simulink model "dcMotor_DiagramBlocks"  (R2018a)
settings: Solver=VariableStepAuto  StartTime=0.0  StopTime=10.0  RelTol=1e-3
libraries: simulink x4
settings Model: Creator=Igor  LastModifiedBy=david

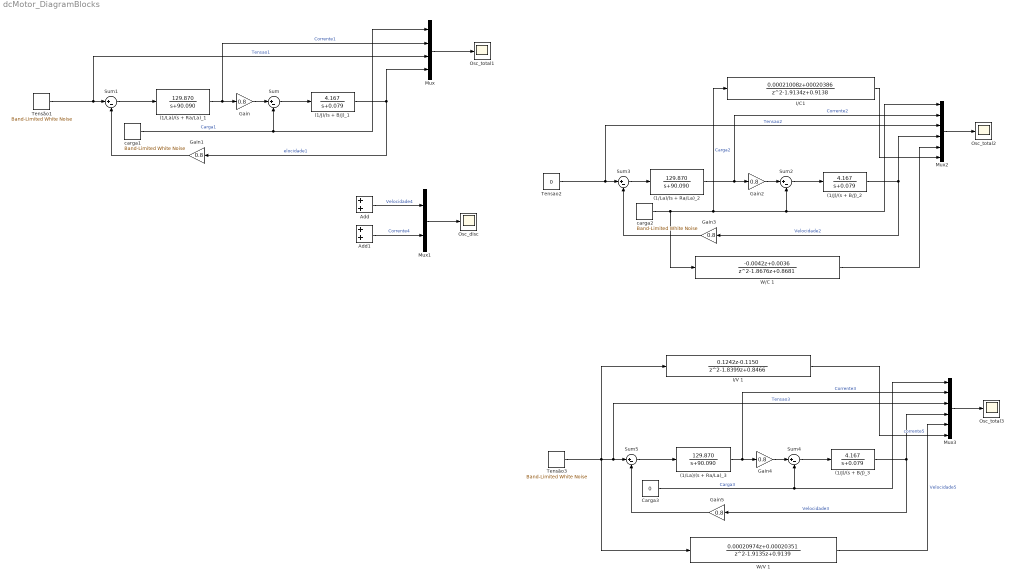
== system dcMotor_DiagramBlocks ==
  (1/J)/(s + B/J)_1 : TransferFcn  Numerator=[4.167]  Denominator=[1 0.079]
  (1/J)/(s + B/J)_2 : TransferFcn  Numerator=[4.167]  Denominator=[1 0.079]
  (1/J)/(s + B/J)_3 : TransferFcn  Numerator=[4.167]  Denominator=[1 0.079]
  (1/La)/(s + Ra/La)_1 : TransferFcn  Numerator=[129.870]  Denominator=[1 90.090 ]
  (1/La)/(s + Ra/La)_2 : TransferFcn  Numerator=[129.870]  Denominator=[1 90.090 ]
  (1/La)/(s + Ra/La)_3 : TransferFcn  Numerator=[129.870]  Denominator=[1 90.090 ]
  Add : Sum
  Add1 : Sum
  Carga3 : Constant  Value=0  SampleTime=0.001
  Gain{,1..5} (6 alike) : Gain  Gain=0.8
  I/C1 : DiscreteTransferFcn  Numerator=[0.00021008 00020386]  Denominator=[1 -1.9134 0.9138]  SampleTime=0.001
  I/V 1 : DiscreteTransferFcn  Numerator=[0.1242 -0.1150]  Denominator=[1 -1.8399 0.8466]  SampleTime=0.001
  Mux : Mux
  Mux1 : Mux  Inputs=2
  Mux2 : Mux  Inputs=6
  Mux3 : Mux  Inputs=6
  Osc_disc : Scope
  Osc_total1 : Scope
  Osc_total2 : Scope
  Osc_total3 : Scope
  Sum{,1..5} (6 alike) : Sum  Inputs=|+-
  Tensao2 : Constant  Value=0  SampleTime=0.001
  "Tensão1 " : simulink/Sources/Band-Limited White Noise  Tag=Tensão  Cov=[10]  Ts=0.001  seed=[23342]
  Tensão3 : simulink/Sources/Band-Limited White Noise  Tag=Tensão  Cov=[10]  Ts=0.001  seed=[23342]
  W/C 1 : DiscreteTransferFcn  Numerator=[ -0.0042 0.0036]  Denominator=[ 1 -1.8676 0.8681 ]  SampleTime=0.001
  W/V 1 : DiscreteTransferFcn  Numerator=[ 0.00020974 0.00020351]  Denominator=[ 1 -1.9135 0.9139 ]  SampleTime=0.001
  carga1 : simulink/Sources/Band-Limited White Noise  Cov=[02]  Ts=0.001  seed=[23341]
  carga2 : simulink/Sources/Band-Limited White Noise  Cov=[02]  Ts=0.001  seed=[23341]
  wires:
  (1/La)/(s + Ra/La)_1/1 -> Mux/2, Gain/1  "Corrente1"
  Sum1/1 -> (1/La)/(s + Ra/La)_1/1
  (1/J)/(s + B/J)_1/1 -> Gain1/1, Mux/4  "elocidade1"
  Gain/1 -> Sum/1
  Sum/1 -> (1/J)/(s + B/J)_1/1
  Gain1/1 -> Sum1/2
  carga1/1 -> Mux/1, Sum/2  "Carga1"
  Mux/1 -> Osc_total1/1
  Add/1 -> Mux1/1  "Velocidade4"
  Add1/1 -> Mux1/2  "Corrente4"
  "Tensão1 "/1 -> Sum1/1, Mux/3  "Tensao1"
  Mux1/1 -> Osc_disc/1
  Mux2/1 -> Osc_total2/1
  Sum3/1 -> (1/La)/(s + Ra/La)_2/1
  carga2/1 -> W/C 1/1, I/C1/1, Mux2/1, Sum2/2  "Carga2"
  Sum2/1 -> (1/J)/(s + B/J)_2/1
  Gain2/1 -> Sum2/1
  Gain3/1 -> Sum3/2
  (1/La)/(s + Ra/La)_2/1 -> Mux2/2, Gain2/1  "Corrente2"
  (1/J)/(s + B/J)_2/1 -> Gain3/1, Mux2/4  "Velocidade2"
  Tensao2/1 -> Sum3/1, Mux2/3  "Tensao2"
  (1/La)/(s + Ra/La)_3/1 -> Mux3/2, Gain4/1  "Corrente3"
  Carga3/1 -> Mux3/1, Sum4/2  "Carga3"
  Gain4/1 -> Sum4/1
  Sum4/1 -> (1/J)/(s + B/J)_3/1
  Gain5/1 -> Sum5/2
  Tensão3/1 -> W/V 1/1, I/V 1/1, Sum5/1, Mux3/3  "Tensao3"
  Sum5/1 -> (1/La)/(s + Ra/La)_3/1
  Mux3/1 -> Osc_total3/1
  (1/J)/(s + B/J)_3/1 -> Gain5/1, Mux3/4  "Velocidade3"
  W/V 1/1 -> Mux3/5  "Velocidade5"
  I/V 1/1 -> Mux3/6  "corrente5"
  W/C 1/1 -> Mux2/5
  I/C1/1 -> Mux2/6
